simulink model "gm_Tx_OFDM"  (R2023a)
settings: Solver=FixedStepAuto  StartTime=0.0  StopTime=inf  RelTol=1e-3  EnableMultiTasking=on
model workspace (MAT data in the model file):
  M_ary = 16
  N = 64
  bit_per_symbol = 4
  fsc = 10000
  fsp = 150000
  stime = 0.0001
libraries: simulink x5, hdlmdlgenlib x4, dspsigops x4, commrandsrc3 x1, dsphdlxfrm2 x1, commdigbbndam3 x1
settings Model: Creator=acer  LastModifiedBy=acer
settings OptimizationCC: BlockReduction=off  ConditionallyExecuteInputs=off  EnhancedBackFolding=on  PassReuseOutputArgsAs=Individual arguments  ZeroExternalMemoryAtStartup=off  ZeroInternalMemoryAtStartup=off  MaxStackSize=64  OptimizeBlockOrder=speed  DifferentSizesBufferReuse=on  OptimizationCustomize=off  EfficientTunableParamExpr=on
settings DebuggingCC: InheritedTsInSrcMsg=none  SingleTaskRateTransMsg=error  ParameterTunabilityLossMsg=error
settings HardwareCC: ProdBitPerPointer=32  ProdBitPerSizeT=32  ProdBitPerPtrDiffT=32  ProdLargestAtomicInteger=Long  ProdLargestAtomicFloat=Double  ProdWordSize=32  ProdHWDeviceType=ARM Compatible->ARM Cortex
settings SFSimCC: MATLABDynamicMemAlloc=off
settings RTWCC: Description=Embedded Coder  SystemTargetFile=ert.tlc  TLCOptions="-aInlineSetEventsForThisBaseRateFcn=TLC_FALSE -aSuppressMultiTaskScheduler=TLC_FALSE  -aRateBasedStepFcn=0"  TemplateMakefile=ert_default_tmf
settings CodeAppCC: ForceParamTrailComments=on  IgnoreCustomStorageClasses=off  OperatorAnnotations=on  SimulinkDataObjDesc=on  SFDataObjDesc=on  InsertBlockDesc=on

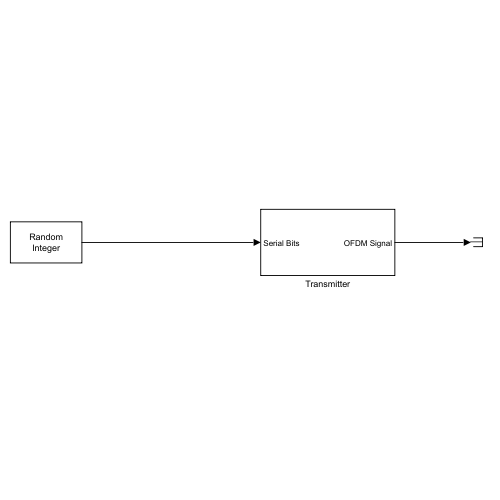
[thumbnail: Simulink's stored preview of the top-level diagram]
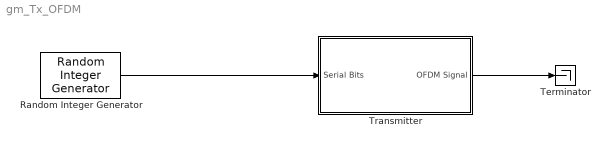
== system gm_Tx_OFDM ==
  Random Integer Generator : commrandsrc3/Random Integer Generator  SetSize=16  SeedSource=Auto  Seed=0  SampleTime=stime  SamplesPerFrame=1  OutputDataType=uint8  SimulateUsing=Interpreted execution
  Terminator : Terminator
  Transmitter : Subsystem
  wires:
  Random Integer Generator/1 -> Transmitter/1(Serial Bits)
  Transmitter/1(OFDM Signal) -> Terminator/1

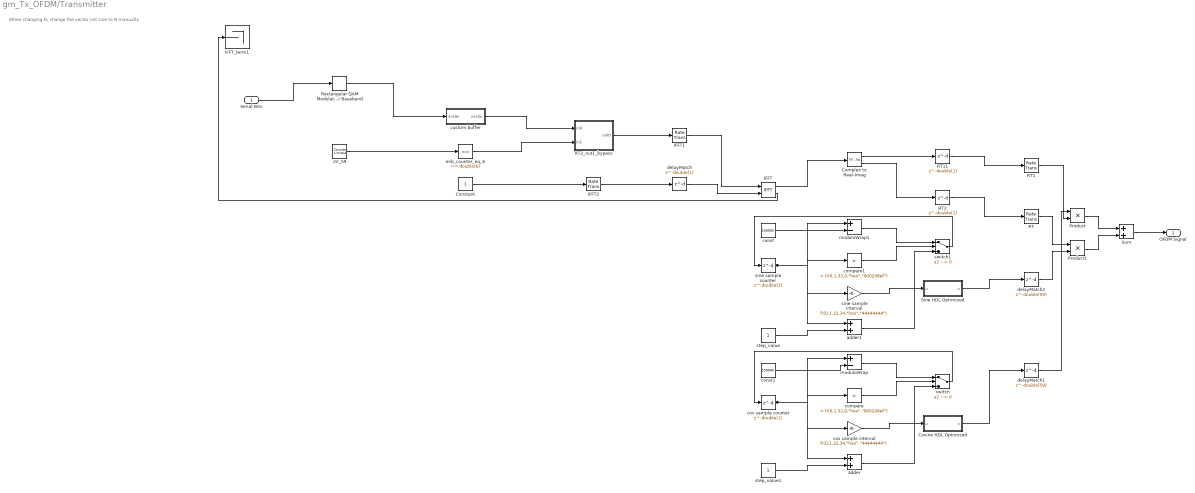
== system gm_Tx_OFDM/Transmitter ==
  note: When changing N, change the vector init size to N manually
  Serial Bits : Inport  OutDataTypeStr=uint8  PortDimensions=1  SampleTime=0.0001
  Complex to Real-Imag : ComplexToRealImag  SampleTime=0.0004
  Constant : Constant  OutDataTypeStr=boolean  SampleTime=6.66666666666667e-06
  Cosine HDL Optimized : Subsystem  mask(Sine and Cosine HDL optimized block){OutputFormula=cos(2*pi*u), NumDataPoints=double(64), TableDataTypeStr=fixdt(0,16,15), SimulateLUTROMDelay=off}
      mask prompts: OutputFormula "Simulink:masks:OutputFormula_MP"; NumDataPoints "HDLShared:hdlshared:CosineHDL_Npts"; TableDataTypeStr "Simulink:blkprm_prompts:TABLE_UNIFIEDDATATYPE"; SimulateLUTROMDelay "HDLShared:hdlshared:CosineHDL_SimulateLUTDelay"
      mask help: Sine and Cosine HDL optimized block using quarter wave symmetry, and HDL friendly settings.
      mask init:
      | NumDataPoints = double(64);
      | OutputFormula = double(2);
      | SampleTime = double(-1);
      | SimulateLUTROMDelay = double(0);
      | TableDataTypeStr = fixdt(0,16,15);
      | curr_blk_name = 'Tx_OFDM/Transmitter/Cosine\nHDL Optimized';
      | sys_name = 'Tx_OFDM/Transmitter';
      mask Help: helpview([docroot '/hdlcoder/helptargets.map'],'SineAndCosineHDL_Optimized');
      mask TypeOptions OutputFormula: sin(2*pi*u) | cos(2*pi*u) | exp(j*2*pi*u) | sin(2*pi*u) and cos(2*pi*u)
      mask Display:
      | port_label('input',1,'u')
      | port_label('output',1,'cos(2*pi*u)')
      | xpos = 0.35;
      | yoffset = 0.5;
      | if ( SimulateLUTROMDelay )
      |   text(xpos,yoffset,'HDL (Z^{-1})','texmode','on')
      | else
      |    text(xpos,yoffset,'HDL')
      | end
  IFFT : dsphdlxfrm2/IFFT  FFTLength=N  Architecture=Streaming Radix 2^2  ComplexMultiplication=Use 4 multipliers and 2 adders  BitReversedOutput=on  BitReversedInput=off  Normalize=on  SimulateUsing=Code generation  RoundingMethod=Floor  ResetInputPort=off  StartOutputPort=off  EndOutputPort=off
  IFFT1 : RateTransition  OutPortSampleTimeOpt=Multiple of input port sample time  OutPortSampleTimeMultiple=60
  IFFT2 : RateTransition  OutPortSampleTimeOpt=Multiple of input port sample time  OutPortSampleTimeMultiple=60
  IFFT_term1 : Terminator
  Product : Product  Inputs=**  OutDataTypeStr=fixdt(1, 33, 29)  SampleTime=6.66666666666667e-06
  Product1 : Product  Inputs=**  OutDataTypeStr=int16  SampleTime=6.66666666666667e-06
  RT : RateTransition  Integrity=off  Deterministic=off  InitialCondition=double(0)  OutPortSampleTimeOpt=Multiple of input port sample time  OutPortSampleTimeMultiple=1/60
  RT1 : RateTransition  Integrity=off  Deterministic=off  InitialCondition=double(0)  OutPortSampleTimeOpt=Multiple of input port sample time  OutPortSampleTimeMultiple=1/60
  RT11 : Delay  DelayLength=double(1)  InitialCondition=0  SampleTime=0.0004
  RT2 : Delay  DelayLength=double(1)  InitialCondition=0  SampleTime=0.0004
  RT2_out1_bypass : Subsystem
  Rectangular QAM Modulator Baseband : commdigbbndam3/Rectangular QAM Modulator Baseband  M=M_ary  InType=Integer  Enc=Gray  Mapping=[0:15]  PowType=Min. distance between symbols  MinDist=2  AvgPow=1  PeakPow=1  Ph=0  outDtype=Fixed-point  outWordLen=16  outUDDataType=sfix(16)  outFracLenMode=Best precision  outFracLen=15  outDataTypeStr=fixdt(1,16)  outLastDataTypeStr=fixdt(1,16)
      settings: LibrarySourceBlock=|
      | commhdldigbbndam/Rectangular QAM
      | Modulator
      | Baseband
  Sine HDL Optimized : Subsystem  mask(Sine and Cosine HDL optimized block){OutputFormula=sin(2*pi*u), NumDataPoints=double(64), TableDataTypeStr=fixdt(0,16,15), SimulateLUTROMDelay=off}
      mask prompts: OutputFormula "Simulink:masks:OutputFormula_MP"; NumDataPoints "HDLShared:hdlshared:CosineHDL_Npts"; TableDataTypeStr "Simulink:blkprm_prompts:TABLE_UNIFIEDDATATYPE"; SimulateLUTROMDelay "HDLShared:hdlshared:CosineHDL_SimulateLUTDelay"
      mask help: Sine and Cosine HDL optimized block using quarter wave symmetry, and HDL friendly settings.
      mask init:
      | NumDataPoints = double(64);
      | OutputFormula = double(1);
      | SampleTime = double(-1);
      | SimulateLUTROMDelay = double(0);
      | TableDataTypeStr = fixdt(0,16,15);
      | curr_blk_name = 'Tx_OFDM/Transmitter/Sine\nHDL Optimized';
      | sys_name = 'Tx_OFDM/Transmitter';
      mask Help: helpview([docroot '/hdlcoder/helptargets.map'],'SineAndCosineHDL_Optimized');
      mask TypeOptions OutputFormula: sin(2*pi*u) | cos(2*pi*u) | exp(j*2*pi*u) | sin(2*pi*u) and cos(2*pi*u)
      mask Display:
      | port_label('input',1,'u')
      | port_label('output',1,'sin(2*pi*u)')
      | xpos = 0.35;
      | yoffset = 0.5;
      | if ( SimulateLUTROMDelay )
      |   text(xpos,yoffset,'HDL (Z^{-1})','texmode','on')
      | else
      |    text(xpos,yoffset,'HDL')
      | end
  Sum : Sum  AccumDataTypeStr=fixdt(1, 64, 29)  OutDataTypeStr=fixdt(1, 64, 29)  SampleTime=6.66666666666667e-06
  adder : Sum  AccumDataTypeStr=int32  OutDataTypeStr=int32  SampleTime=6.66666666666667e-06
  adder1 : Sum  AccumDataTypeStr=int32  OutDataTypeStr=int32  SampleTime=6.66666666666667e-06
  compare : simulink/Logic and Bit Operations/Compare To Constant  relop=>  const="fi(0,1,32,0,\"hex\",\"000249ef\")"  OutDataTypeStr=boolean
  compare1 : simulink/Logic and Bit Operations/Compare To Constant  relop=>  const="fi(0,1,32,0,\"hex\",\"000249ef\")"  OutDataTypeStr=boolean
  const : Constant  Value=150000  VectorParams1D=off  OutDataTypeStr=int32  SampleTime=6.66666666666667e-06
  const1 : Constant  Value=150000  VectorParams1D=off  OutDataTypeStr=int32  SampleTime=6.66666666666667e-06
  cos sample counter : Delay  DelayLength=double(1)  InitialCondition=0  SampleTime=6.66666666666667e-06
  cos sample interval : Gain  Gain="fi(0,1,32,34,\"hex\",\"44444444\")"  ParamDataTypeStr=fixdt(1, 32, 34)  OutDataTypeStr=fixdt(1, 64, 34)  SampleTime=6.66666666666667e-06
  ctr_59 : simulink/Sources/Counter Limited  uplimit=double(59)  tsamp=6.66666666666667e-06
  custom buffer : Subsystem
  delayMatch : Delay  DelayLength=double(1)  InitialCondition=0  SampleTime=0.0004
  delayMatch1 : Delay  DelayLength=double(59)  InitialCondition=0  SampleTime=6.66666666666667e-06
  delayMatch2 : Delay  DelayLength=double(59)  InitialCondition=0  SampleTime=6.66666666666667e-06
  enb_counter_eq_6 : simulink/Logic and Bit Operations/Compare To Constant  relop===  const=double(6)  OutDataTypeStr=boolean
  moduloWrap : Sum  Inputs=+-  AccumDataTypeStr=int32  OutDataTypeStr=int32  SampleTime=6.66666666666667e-06
  moduloWrap1 : Sum  Inputs=+-  AccumDataTypeStr=int32  OutDataTypeStr=int32  SampleTime=6.66666666666667e-06
  sine sample counter : Delay  DelayLength=double(1)  InitialCondition=0  SampleTime=6.66666666666667e-06
  sine sample interval : Gain  Gain="fi(0,1,32,34,\"hex\",\"44444444\")"  ParamDataTypeStr=fixdt(1, 32, 34)  OutDataTypeStr=fixdt(1, 64, 34)  SampleTime=6.66666666666667e-06
  step_value : Constant  VectorParams1D=off  OutDataTypeStr=int32  SampleTime=6.66666666666667e-06
  step_value1 : Constant  VectorParams1D=off  OutDataTypeStr=int32  SampleTime=6.66666666666667e-06
  switch : Switch  Criteria=u2 ~= 0  Threshold=double(0)  OutDataTypeStr=int32  SampleTime=6.66666666666667e-06  SaturateOnIntegerOverflow=off  InputSameDT=off
  switch1 : Switch  Criteria=u2 ~= 0  Threshold=double(0)  OutDataTypeStr=int32  SampleTime=6.66666666666667e-06  SaturateOnIntegerOverflow=off  InputSameDT=off
  OFDM Signal : Outport  SampleTime=6.66666666666667e-06
  wires:
  Serial Bits/1 -> Rectangular QAM Modulator Baseband/1
  IFFT/1 -> Complex to Real-Imag/1
  IFFT/2 -> IFFT_term1/1
  Rectangular QAM Modulator Baseband/1 -> custom buffer/1(scalar)
  Sum/1 -> OFDM Signal/1
  cos sample counter/1 -> cos sample interval/1, compare/1, moduloWrap/1, adder/1
  sine sample counter/1 -> sine sample interval/1, compare1/1, moduloWrap1/1, adder1/1
  RT/1 -> Product1/1
  RT1/1 -> Product/2
  RT11/1 -> RT1/1
  RT2/1 -> RT/1
  sine sample interval/1 -> Sine HDL Optimized/1(u)
  delayMatch2/1 -> Product1/2
  Product1/1 -> Sum/2
  Product/1 -> Sum/1
  cos sample interval/1 -> Cosine HDL Optimized/1(u)
  delayMatch1/1 -> Product/1
  const/1 -> moduloWrap1/2
  step_value/1 -> adder1/2
  const1/1 -> moduloWrap/2
  step_value1/1 -> adder/2
  Complex to Real-Imag/1 -> RT11/1
  Complex to Real-Imag/2 -> RT2/1
  custom buffer/1(vector) -> RT2_out1_bypass/1(in0)
  IFFT1/1 -> IFFT/1
  delayMatch/1 -> IFFT/2
  Constant/1 -> IFFT2/1
  RT2_out1_bypass/1(out0) -> IFFT1/1
  IFFT2/1 -> delayMatch/1
  Cosine HDL Optimized/1(x) -> delayMatch1/1
  Sine HDL Optimized/1(x) -> delayMatch2/1
  switch1/1 -> sine sample counter/1
  adder1/1 -> switch1/3
  compare1/1 -> switch1/2
  moduloWrap1/1 -> switch1/1
  switch/1 -> cos sample counter/1
  adder/1 -> switch/3
  compare/1 -> switch/2
  moduloWrap/1 -> switch/1
  enb_counter_eq_6/1 -> RT2_out1_bypass/2(in1)
  ctr_59/1 -> enb_counter_eq_6/1

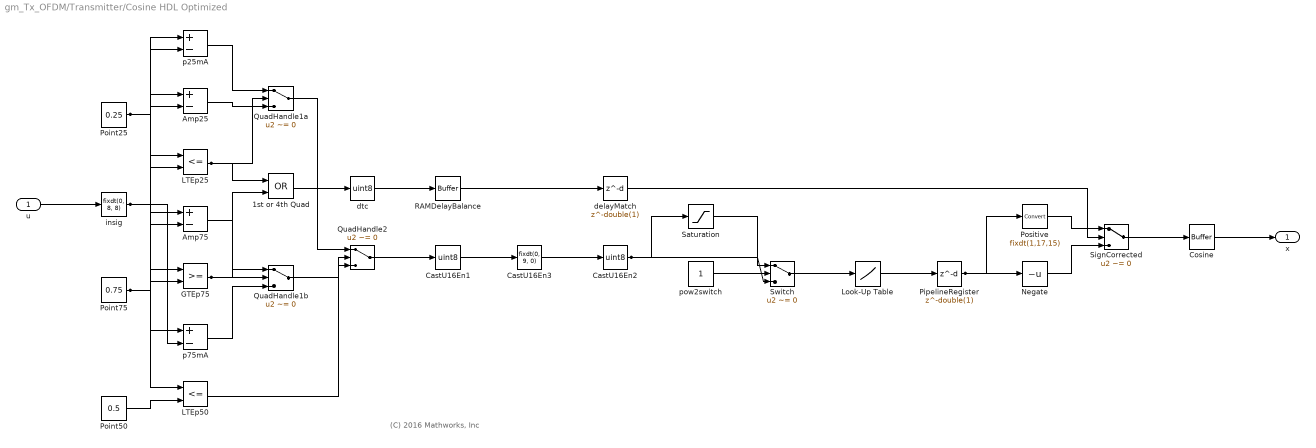
== system gm_Tx_OFDM/Transmitter/Cosine HDL Optimized ==
  note: (C) 2016 Mathworks, Inc
  u : Inport  OutDataTypeStr=fixdt(1,64,34,'DataTypeOverride', 'Off')  SampleTime=6.66666666666667e-06
  1st or 4th Quad : Logic  Operator=OR  AllPortsSameDT=off  OutDataTypeStr=boolean  SampleTime=6.66666666666667e-06
  Amp25 : Sum  Inputs=+-  AccumDataTypeStr=fixdt(1, 32, 17)  OutDataTypeStr=fixdt(0, 32, 17)  SampleTime=6.66666666666667e-06
  Amp75 : Sum  Inputs=+-  AccumDataTypeStr=fixdt(1, 32, 17)  OutDataTypeStr=fixdt(0, 32, 17)  SampleTime=6.66666666666667e-06
  CastU16En1 : DataTypeConversion  OutDataTypeStr=uint8  ConvertRealWorld=Stored Integer (SI)  SampleTime=6.66666666666667e-06  SaturateOnIntegerOverflow=off  RndMeth=Floor
  CastU16En2 : DataTypeConversion  OutDataTypeStr=uint8  ConvertRealWorld=Stored Integer (SI)  SampleTime=6.66666666666667e-06  RndMeth=Floor
  CastU16En3 : DataTypeConversion  OutDataTypeStr=fixdt(0, 9, 0)  SampleTime=6.66666666666667e-06  SaturateOnIntegerOverflow=off  RndMeth=Floor
  Cosine : hdlmdlgenlib/Buffer
  GTEp75 : RelationalOperator  OutDataTypeStr=boolean  SampleTime=6.66666666666667e-06  InputSameDT=off
  LTEp25 : RelationalOperator  Operator=<=  OutDataTypeStr=boolean  SampleTime=6.66666666666667e-06  InputSameDT=off
  LTEp50 : RelationalOperator  Operator=<=  OutDataTypeStr=boolean  SampleTime=6.66666666666667e-06  InputSameDT=off
  Look-Up Table : Lookup_n-D  NumberOfTableDimensions=1  BreakpointsForDimension1="fi(\"numerictype\",numerictype(0,8,0),\"fimath\",fimath(\"RoundingMethod\", \"Floor\",\"OverflowAction\", \"Wrap\",\"ProductMode\",\"FullPrecision\",\"SumMode\",\"FullPrecision\"),\"Value\",\"[0 1 2 3 4 5 6 7 8 9 10 11 12 13 14 15 16 17 18 19 20 21 22 23 24 25 26 27 28 29 30 31 32 33 34 35 36 37 38 39 40 41 42 43 44 45 46 47 48 49 50 51 52 53 54 55 56 57 58 59 60 61 62 63]\")"  Table="reshape(fi(\"numerictype\",numerictype(1,17,15),\"fimath\",fimath(\"RoundingMethod\", \"Floor\",\"OverflowAction\", \"Wrap\",\"ProductMode\",\"FullPrecision\",\"SumMode\",\"FullPrecision\"),\"Value\",\"[0;0.0245361328125;0.049072265625;0.073577880859375;0.0980224609375;0.122406005859375;0.146728515625;0.17095947265625;0.195098876953125;0.2191162109375;0.24298095703125;0.2667236328125;0.290283203125;0.313690185546875;0.336883544921875;0.359893798828125;0.3826904296875;0.405242919921875;0.42755126953125;0.449615478515625;0.471405029296875;0.492889404296875;0.51409912109375;0.535003662109375;0.555572509765625;0.5758056640625;0.595703125;0.615234375;0.6343994140625;0.653167724609375;0.67156982421875;0.689544677734375;0.70709228515625;0.7242431640625;0.740936279296875;0.7572021484375;0.77301025390625;0.788360595703125;0.80322265625;0.817596435546875;0.83148193359375;0.8448486328125;0.85772705078125;0.870086669921875;0.881927490234375;0.893218994140625;0.90399169921875;0.914215087890625;0.92388916015625;0.9329833984375;0.941558837890625;0.94952392578125;0.956939697265625;0.963775634765625;0.97003173828125;0.9757080078125;0.98077392578125;0.98529052734375;0.989166259765625;0.99249267578125;0.99517822265625;0.997283935546875;0.998809814453125;0.99969482421875]\"), [1  64])"  InterpMethod=Flat  ExtrapMethod=Clip  DiagnosticForOutOfRangeInput=Error  SampleTime=6.66666666666667e-06  OutDataTypeStr=fixdt(1, 17, 15)
  Negate : UnaryMinus  SampleTime=6.66666666666667e-06
  PipelineRegister : Delay  DelayLength=double(1)  InitialCondition=0  SampleTime=6.66666666666667e-06
  Point25 : Constant  Value=0.25  OutDataTypeStr=fixdt(0, 17, 17)  SampleTime=6.66666666666667e-06
  Point50 : Constant  Value=0.5  OutDataTypeStr=fixdt(0, 17, 17)  SampleTime=6.66666666666667e-06
  Point75 : Constant  Value=0.75  OutDataTypeStr=fixdt(0, 17, 17)  SampleTime=6.66666666666667e-06
  Positive : DataTypeConversion  OutDataTypeStr=fixdt(1,17,15)
  QuadHandle1a : Switch  Criteria=u2 ~= 0  Threshold=double(0)  OutDataTypeStr=fixdt(0, 32, 17)  SampleTime=6.66666666666667e-06  SaturateOnIntegerOverflow=off  InputSameDT=off
  QuadHandle1b : Switch  Criteria=u2 ~= 0  Threshold=double(0)  OutDataTypeStr=fixdt(0, 32, 17)  SampleTime=6.66666666666667e-06  SaturateOnIntegerOverflow=off  InputSameDT=off
  QuadHandle2 : Switch  Criteria=u2 ~= 0  Threshold=double(0)  OutDataTypeStr=fixdt(0, 8, 8)  SampleTime=6.66666666666667e-06  InputSameDT=off
  RAMDelayBalance : hdlmdlgenlib/Buffer
  Saturation : Saturate  UpperLimit="fi(0,0,8,0,\"hex\",\"3f\")"  LowerLimit="fi(0,0,8,0,\"hex\",\"00\")"  SampleTime=6.66666666666667e-06  OutDataTypeStr=uint8
  SignCorrected : Switch  Criteria=u2 ~= 0  Threshold=double(0)  OutDataTypeStr=fixdt(1, 17, 15)  SampleTime=6.66666666666667e-06  SaturateOnIntegerOverflow=off  InputSameDT=off
  Switch : Switch  Criteria=u2 ~= 0  Threshold=double(0)  OutDataTypeStr=uint8  SampleTime=6.66666666666667e-06  SaturateOnIntegerOverflow=off  InputSameDT=off
  delayMatch : Delay  DelayLength=double(1)  InitialCondition=0  SampleTime=6.66666666666667e-06
  dtc : DataTypeConversion  OutDataTypeStr=uint8  ConvertRealWorld=Stored Integer (SI)  SampleTime=6.66666666666667e-06  SaturateOnIntegerOverflow=off  RndMeth=Floor
  insig : DataTypeConversion  OutDataTypeStr=fixdt(0, 8, 8)  SampleTime=6.66666666666667e-06  SaturateOnIntegerOverflow=off  RndMeth=Floor
  p25mA : Sum  Inputs=+-  AccumDataTypeStr=fixdt(1, 32, 17)  OutDataTypeStr=fixdt(0, 32, 17)  SampleTime=6.66666666666667e-06
  p75mA : Sum  Inputs=+-  AccumDataTypeStr=fixdt(1, 32, 17)  OutDataTypeStr=fixdt(0, 32, 17)  SampleTime=6.66666666666667e-06
  pow2switch : Constant  OutDataTypeStr=boolean  SampleTime=6.66666666666667e-06
  x : Outport  SampleTime=6.66666666666667e-06
  wires:
  Cosine/1 -> x/1
  dtc/1 -> RAMDelayBalance/1
  Amp25/1 -> QuadHandle1a/3
  Amp75/1 -> QuadHandle1b/1
  CastU16En1/1 -> CastU16En3/1
  CastU16En2/1 -> Switch/3, Saturation/1
  CastU16En3/1 -> CastU16En2/1
  GTEp75/1 -> QuadHandle1b/2, 1st or 4th Quad/2
  LTEp25/1 -> QuadHandle1a/2, 1st or 4th Quad/1
  LTEp50/1 -> QuadHandle2/2
  PipelineRegister/1 -> Positive/1, Negate/1
  Negate/1 -> SignCorrected/3
  Point25/1 -> p25mA/1, LTEp25/2, Amp25/2
  Point50/1 -> LTEp50/2
  Point75/1 -> p75mA/1, GTEp75/2, Amp75/2
  Positive/1 -> SignCorrected/1
  QuadHandle1a/1 -> QuadHandle2/1
  QuadHandle1b/1 -> QuadHandle2/3
  QuadHandle2/1 -> CastU16En1/1
  delayMatch/1 -> SignCorrected/2
  Saturation/1 -> Switch/1
  SignCorrected/1 -> Cosine/1
  Switch/1 -> Look-Up Table/1
  insig/1 -> p75mA/2, p25mA/2, LTEp50/1, LTEp25/1, GTEp75/1, Amp75/1, Amp25/1
  p25mA/1 -> QuadHandle1a/1
  p75mA/1 -> QuadHandle1b/3
  pow2switch/1 -> Switch/2
  1st or 4th Quad/1 -> dtc/1
  u/1 -> insig/1
  RAMDelayBalance/1 -> delayMatch/1
  Look-Up Table/1 -> PipelineRegister/1

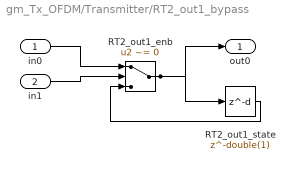
== system gm_Tx_OFDM/Transmitter/RT2_out1_bypass ==
  in0 : Inport  OutDataTypeStr=fixdt(1,16,14,'DataTypeOverride', 'Off')  PortDimensions=[64]  SampleTime=6.66666666666667e-06
      settings: SignalType=complex
  in1 : Inport  Port=2  OutDataTypeStr=boolean  SampleTime=6.66666666666667e-06
  RT2_out1_enb : Switch  Criteria=u2 ~= 0  Threshold=double(0)  OutDataTypeStr=fixdt(1, 16, 14)  SampleTime=6.66666666666667e-06  SaturateOnIntegerOverflow=off  InputSameDT=off
  RT2_out1_state : Delay  DelayLength=double(1)  InitialCondition=0  SampleTime=6.66666666666667e-06
  out0 : Outport  OutDataTypeStr=fixdt(1, 16, 14)  PortDimensions=[64]  SampleTime=6.66666666666667e-06
      settings: SignalType=complex
  wires:
  RT2_out1_enb/1 -> out0/1, RT2_out1_state/1
  in0/1 -> RT2_out1_enb/1
  in1/1 -> RT2_out1_enb/2
  RT2_out1_state/1 -> RT2_out1_enb/3

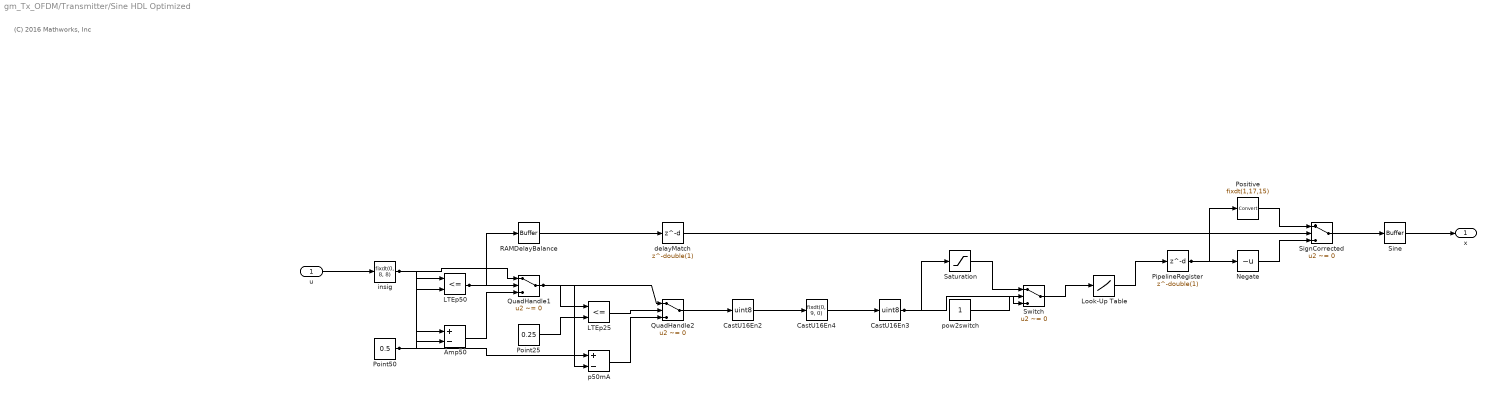
== system gm_Tx_OFDM/Transmitter/Sine HDL Optimized ==
  note: (C) 2016 Mathworks, Inc
  u : Inport  OutDataTypeStr=fixdt(1,64,34,'DataTypeOverride', 'Off')  SampleTime=6.66666666666667e-06
  Amp50 : Sum  Inputs=+-  AccumDataTypeStr=fixdt(1, 32, 17)  OutDataTypeStr=fixdt(0, 32, 17)  SampleTime=6.66666666666667e-06
  CastU16En2 : DataTypeConversion  OutDataTypeStr=uint8  ConvertRealWorld=Stored Integer (SI)  SampleTime=6.66666666666667e-06  SaturateOnIntegerOverflow=off  RndMeth=Floor
  CastU16En3 : DataTypeConversion  OutDataTypeStr=uint8  ConvertRealWorld=Stored Integer (SI)  SampleTime=6.66666666666667e-06  RndMeth=Floor
  CastU16En4 : DataTypeConversion  OutDataTypeStr=fixdt(0, 9, 0)  SampleTime=6.66666666666667e-06  SaturateOnIntegerOverflow=off  RndMeth=Floor
  LTEp25 : RelationalOperator  Operator=<=  OutDataTypeStr=boolean  SampleTime=6.66666666666667e-06  InputSameDT=off
  LTEp50 : RelationalOperator  Operator=<=  OutDataTypeStr=boolean  SampleTime=6.66666666666667e-06  InputSameDT=off
  Look-Up Table : Lookup_n-D  NumberOfTableDimensions=1  BreakpointsForDimension1="fi(\"numerictype\",numerictype(0,8,0),\"fimath\",fimath(\"RoundingMethod\", \"Floor\",\"OverflowAction\", \"Wrap\",\"ProductMode\",\"FullPrecision\",\"SumMode\",\"FullPrecision\"),\"Value\",\"[0 1 2 3 4 5 6 7 8 9 10 11 12 13 14 15 16 17 18 19 20 21 22 23 24 25 26 27 28 29 30 31 32 33 34 35 36 37 38 39 40 41 42 43 44 45 46 47 48 49 50 51 52 53 54 55 56 57 58 59 60 61 62 63]\")"  Table="reshape(fi(\"numerictype\",numerictype(1,17,15),\"fimath\",fimath(\"RoundingMethod\", \"Floor\",\"OverflowAction\", \"Wrap\",\"ProductMode\",\"FullPrecision\",\"SumMode\",\"FullPrecision\"),\"Value\",\"[0;0.0245361328125;0.049072265625;0.073577880859375;0.0980224609375;0.122406005859375;0.146728515625;0.17095947265625;0.195098876953125;0.2191162109375;0.24298095703125;0.2667236328125;0.290283203125;0.313690185546875;0.336883544921875;0.359893798828125;0.3826904296875;0.405242919921875;0.42755126953125;0.449615478515625;0.471405029296875;0.492889404296875;0.51409912109375;0.535003662109375;0.555572509765625;0.5758056640625;0.595703125;0.615234375;0.6343994140625;0.653167724609375;0.67156982421875;0.689544677734375;0.70709228515625;0.7242431640625;0.740936279296875;0.7572021484375;0.77301025390625;0.788360595703125;0.80322265625;0.817596435546875;0.83148193359375;0.8448486328125;0.85772705078125;0.870086669921875;0.881927490234375;0.893218994140625;0.90399169921875;0.914215087890625;0.92388916015625;0.9329833984375;0.941558837890625;0.94952392578125;0.956939697265625;0.963775634765625;0.97003173828125;0.9757080078125;0.98077392578125;0.98529052734375;0.989166259765625;0.99249267578125;0.99517822265625;0.997283935546875;0.998809814453125;0.99969482421875]\"), [1  64])"  InterpMethod=Flat  ExtrapMethod=Clip  DiagnosticForOutOfRangeInput=Error  SampleTime=6.66666666666667e-06  OutDataTypeStr=fixdt(1, 17, 15)
  Negate : UnaryMinus  SampleTime=6.66666666666667e-06
  PipelineRegister : Delay  DelayLength=double(1)  InitialCondition=0  SampleTime=6.66666666666667e-06
  Point25 : Constant  Value=0.25  OutDataTypeStr=fixdt(0, 17, 17)  SampleTime=6.66666666666667e-06
  Point50 : Constant  Value=0.5  OutDataTypeStr=fixdt(0, 17, 17)  SampleTime=6.66666666666667e-06
  Positive : DataTypeConversion  OutDataTypeStr=fixdt(1,17,15)
  QuadHandle1 : Switch  Criteria=u2 ~= 0  Threshold=double(0)  OutDataTypeStr=fixdt(0, 32, 17)  SampleTime=6.66666666666667e-06  SaturateOnIntegerOverflow=off  InputSameDT=off
  QuadHandle2 : Switch  Criteria=u2 ~= 0  Threshold=double(0)  OutDataTypeStr=fixdt(0, 8, 8)  SampleTime=6.66666666666667e-06  SaturateOnIntegerOverflow=off  InputSameDT=off
  RAMDelayBalance : hdlmdlgenlib/Buffer
  Saturation : Saturate  UpperLimit="fi(0,0,8,0,\"hex\",\"3f\")"  LowerLimit="fi(0,0,8,0,\"hex\",\"00\")"  SampleTime=6.66666666666667e-06  OutDataTypeStr=uint8
  SignCorrected : Switch  Criteria=u2 ~= 0  Threshold=double(0)  OutDataTypeStr=fixdt(1, 17, 15)  SampleTime=6.66666666666667e-06  SaturateOnIntegerOverflow=off  InputSameDT=off
  Sine : hdlmdlgenlib/Buffer
  Switch : Switch  Criteria=u2 ~= 0  Threshold=double(0)  OutDataTypeStr=uint8  SampleTime=6.66666666666667e-06  SaturateOnIntegerOverflow=off  InputSameDT=off
  delayMatch : Delay  DelayLength=double(1)  InitialCondition=0  SampleTime=6.66666666666667e-06
  insig : DataTypeConversion  OutDataTypeStr=fixdt(0, 8, 8)  SampleTime=6.66666666666667e-06  SaturateOnIntegerOverflow=off  RndMeth=Floor
  p50mA : Sum  Inputs=+-  AccumDataTypeStr=fixdt(0, 32, 17)  OutDataTypeStr=fixdt(0, 32, 17)  SampleTime=6.66666666666667e-06
  pow2switch : Constant  OutDataTypeStr=boolean  SampleTime=6.66666666666667e-06
  x : Outport  SampleTime=6.66666666666667e-06
  wires:
  Sine/1 -> x/1
  Amp50/1 -> QuadHandle1/3
  CastU16En2/1 -> CastU16En4/1
  CastU16En3/1 -> Switch/3, Saturation/1
  CastU16En4/1 -> CastU16En3/1
  LTEp25/1 -> QuadHandle2/2
  LTEp50/1 -> QuadHandle1/2, RAMDelayBalance/1
  PipelineRegister/1 -> Positive/1, Negate/1
  Negate/1 -> SignCorrected/3
  Point25/1 -> LTEp25/2
  Point50/1 -> p50mA/1, LTEp50/2, Amp50/2
  Positive/1 -> SignCorrected/1
  QuadHandle1/1 -> p50mA/2, QuadHandle2/1, LTEp25/1
  QuadHandle2/1 -> CastU16En2/1
  delayMatch/1 -> SignCorrected/2
  Saturation/1 -> Switch/1
  SignCorrected/1 -> Sine/1
  Switch/1 -> Look-Up Table/1
  insig/1 -> QuadHandle1/1, LTEp50/1, Amp50/1
  p50mA/1 -> QuadHandle2/3
  pow2switch/1 -> Switch/2
  u/1 -> insig/1
  RAMDelayBalance/1 -> delayMatch/1
  Look-Up Table/1 -> PipelineRegister/1

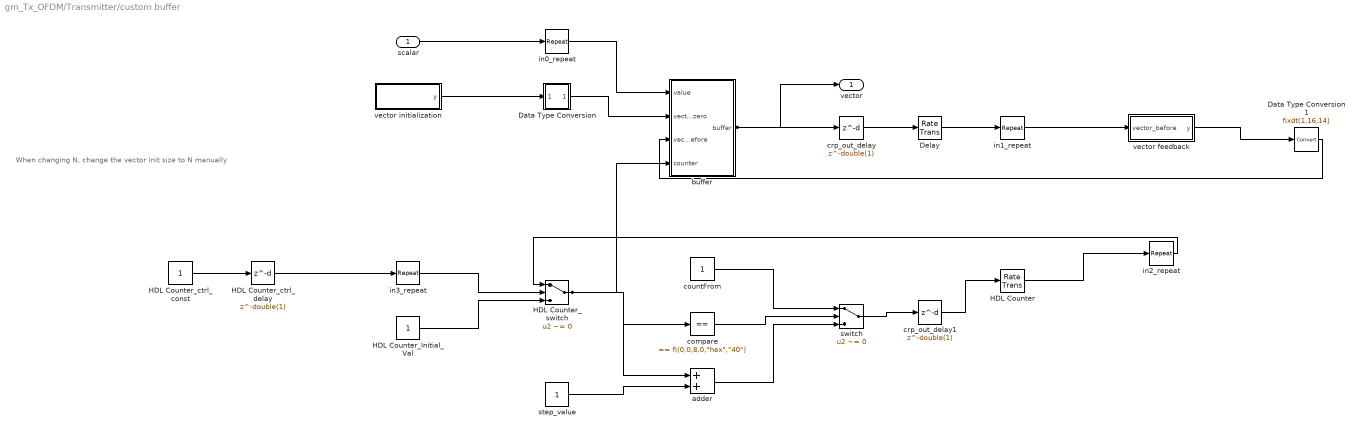
== system gm_Tx_OFDM/Transmitter/custom buffer ==
  note: When changing N, change the vector init size to N manually
  scalar : Inport  OutDataTypeStr=fixdt(1, 16, 13)  PortDimensions=1  SampleTime=0.0001
      settings: SignalType=complex
  Data Type Conversion : Subsystem
      mask Display: disp('NFP\nconv');
  Data Type Conversion1 : DataTypeConversion  OutDataTypeStr=fixdt(1,16,14)
  Delay : RateTransition  OutPortSampleTimeOpt=Multiple of input port sample time  OutPortSampleTimeMultiple=15
  HDL Counter : RateTransition  OutPortSampleTimeOpt=Multiple of input port sample time  OutPortSampleTimeMultiple=15
  HDL Counter_Initial_Val : Constant  OutDataTypeStr=uint8  SampleTime=6.66666666666667e-06
  HDL Counter_ctrl_const : Constant  OutDataTypeStr=boolean  SampleTime=0.0001
  HDL Counter_ctrl_delay : Delay  DelayLength=double(1)  InitialCondition=0  SampleTime=0.0001
  HDL Counter_switch : Switch  Criteria=u2 ~= 0  Threshold=double(0)  OutDataTypeStr=uint8  SampleTime=6.66666666666667e-06  SaturateOnIntegerOverflow=off  InputSameDT=off
  adder : Sum  AccumDataTypeStr=uint8  OutDataTypeStr=uint8  SampleTime=6.66666666666667e-06
  buffer : Subsystem
  compare : simulink/Logic and Bit Operations/Compare To Constant  relop===  const="fi(0,0,8,0,\"hex\",\"40\")"  OutDataTypeStr=boolean
  countFrom : Constant  VectorParams1D=off  OutDataTypeStr=uint8  SampleTime=6.66666666666667e-06
  crp_out_delay : Delay  DelayLength=double(1)  InitialCondition=0  SampleTime=6.66666666666667e-06
  crp_out_delay1 : Delay  DelayLength=double(1)  InitialCondition=0  SampleTime=6.66666666666667e-06
  in0_repeat : dspsigops/Repeat  FactorSource=Dialog parameter  N=double(15)  Nmax=16  RateOptions=Allow multirate processing  ic=0  mode=Unused parameter value
  in1_repeat : dspsigops/Repeat  FactorSource=Dialog parameter  N=double(15)  Nmax=16  RateOptions=Allow multirate processing  ic=0  mode=Unused parameter value
  in2_repeat : dspsigops/Repeat  FactorSource=Dialog parameter  N=double(15)  Nmax=16  RateOptions=Allow multirate processing  ic=0  mode=Unused parameter value
  in3_repeat : dspsigops/Repeat  FactorSource=Dialog parameter  N=double(15)  Nmax=16  RateOptions=Allow multirate processing  ic=0  mode=Unused parameter value
  step_value : Constant  VectorParams1D=off  OutDataTypeStr=uint8  SampleTime=6.66666666666667e-06
  switch : Switch  Criteria=u2 ~= 0  Threshold=double(0)  OutDataTypeStr=uint8  SampleTime=6.66666666666667e-06  SaturateOnIntegerOverflow=off  InputSameDT=off
  vector feedback : Subsystem
  vector initialization : Subsystem
  vector : Outport  SampleTime=6.66666666666667e-06
  wires:
  HDL Counter_ctrl_delay/1 -> in3_repeat/1
  HDL Counter_ctrl_const/1 -> HDL Counter_ctrl_delay/1
  buffer/1(buffer) -> vector/1, crp_out_delay/1
  in0_repeat/1 -> buffer/1(value)
  in3_repeat/1 -> HDL Counter_switch/2
  scalar/1 -> in0_repeat/1
  HDL Counter/1 -> in2_repeat/1
  in2_repeat/1 -> HDL Counter_switch/1
  Delay/1 -> in1_repeat/1
  in1_repeat/1 -> vector feedback/1(vector_before)
  crp_out_delay/1 -> Delay/1
  crp_out_delay1/1 -> HDL Counter/1
  vector feedback/1(y) -> Data Type Conversion1/1
  Data Type Conversion1/1 -> buffer/3(vector_before)
  countFrom/1 -> switch/1
  step_value/1 -> adder/2
  adder/1 -> switch/3
  switch/1 -> crp_out_delay1/1
  compare/1 -> switch/2
  HDL Counter_Initial_Val/1 -> HDL Counter_switch/3
  HDL Counter_switch/1 -> compare/1, adder/1, buffer/4(counter)
  vector initialization/1(y) -> Data Type Conversion/1(In1)
  Data Type Conversion/1(Out1) -> buffer/2(vector_zero)

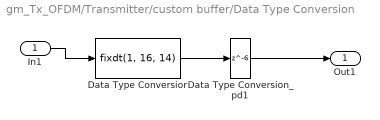
== system gm_Tx_OFDM/Transmitter/custom buffer/Data Type Conversion ==
  In1 : Inport
  Data Type Conversion : DataTypeConversion  OutDataTypeStr=fixdt(1, 16, 14)  SampleTime=6.66666666666667e-06  SaturateOnIntegerOverflow=off  RndMeth=Floor
  Data Type Conversion_pd1 : Delay  DelayLength=6
  Out1 : Outport
  wires:
  In1/1 -> Data Type Conversion/1
  Data Type Conversion/1 -> Data Type Conversion_pd1/1
  Data Type Conversion_pd1/1 -> Out1/1

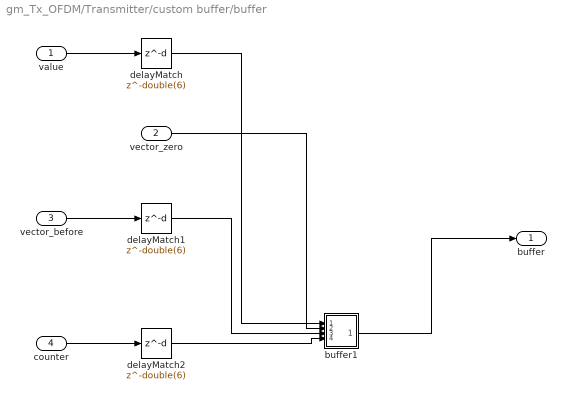
== system gm_Tx_OFDM/Transmitter/custom buffer/buffer ==
  value : Inport  OutDataTypeStr=fixdt(1, 16, 13)  PortDimensions=1  SampleTime=6.66666666666667e-06
      settings: SignalType=complex
  vector_zero : Inport  Port=2  OutDataTypeStr=fixdt(1, 16, 14)  PortDimensions=[64]  SampleTime=6.66666666666667e-06
      settings: SignalType=complex
  vector_before : Inport  Port=3  OutDataTypeStr=fixdt(1, 16, 14)  PortDimensions=[64]  SampleTime=6.66666666666667e-06
      settings: SignalType=complex
  counter : Inport  Port=4  OutDataTypeStr=uint8  PortDimensions=1  SampleTime=6.66666666666667e-06
  buffer1 : MATLAB Function  TreatAsAtomicUnit=on
  delayMatch : Delay  DelayLength=double(6)  InitialCondition=0  SampleTime=6.66666666666667e-06
  delayMatch1 : Delay  DelayLength=double(6)  InitialCondition=0  SampleTime=6.66666666666667e-06
  delayMatch2 : Delay  DelayLength=double(6)  InitialCondition=0  SampleTime=6.66666666666667e-06
  buffer : Outport  SampleTime=6.66666666666667e-06
  wires:
  buffer1/1(buffer) -> buffer/1
  delayMatch/1 -> buffer1/1(value)
  delayMatch1/1 -> buffer1/3(vector_before)
  delayMatch2/1 -> buffer1/4(counter)
  value/1 -> delayMatch/1
  vector_zero/1 -> buffer1/2(vector_zero)
  vector_before/1 -> delayMatch1/1
  counter/1 -> delayMatch2/1

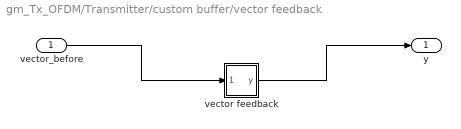
== system gm_Tx_OFDM/Transmitter/custom buffer/vector feedback ==
  vector_before : Inport  OutDataTypeStr=fixdt(1, 16, 14)  PortDimensions=[64]  SampleTime=6.66666666666667e-06
      settings: SignalType=complex
  vector feedback : MATLAB Function  TreatAsAtomicUnit=on
  y : Outport  SampleTime=6.66666666666667e-06  VectorParamsAs1DForOutWhenUnconnected=off
  wires:
  vector feedback/1(y) -> y/1
  vector_before/1 -> vector feedback/1(vector_before)

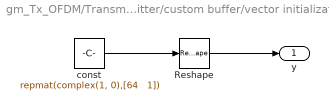
== system gm_Tx_OFDM/Transmitter/custom buffer/vector initialization ==
  Reshape : Reshape
  const : Constant  Value="repmat(complex(1, 0),[64   1])"  VectorParams1D=off  OutDataTypeStr=double  SampleTime=6.66666666666667e-06
  y : Outport  SampleTime=6.66666666666667e-06  VectorParamsAs1DForOutWhenUnconnected=off
  wires:
  Reshape/1 -> y/1
  const/1 -> Reshape/1

== matlab function gm_Tx_OFDM/Transmitter/custom buffer/buffer/buffer1 ==
  data: value input; vector_zero input; vector_before input; counter input; buffer output
function buffer = fcn(value, vector_zero, vector_before, counter)
%#codegen
if(counter == 0)
    buffer = vector_zero;
else
    buffer = vector_before;
end

buffer(counter) = value;

== matlab function gm_Tx_OFDM/Transmitter/custom buffer/vector feedback/vector feedback ==
  data: y output; vector_before input
function y = fcn(vector_before)
%#codegen

y = complex(vector_before);
